simulink model "Diff_eqn"  (R2017b)
settings: Solver=VariableStepAuto  StartTime=0.0  StopTime=10.0  RelTol=1e-3
InitFcn:
  | A=2;
  |  B=4;
  |  C=200;
  | n=25;
  | Amp=10
undefined symbols (not defined in the file or in its folder): function_pulse
settings Model: Creator=ng8a07e  LastModifiedBy=ng8a07e

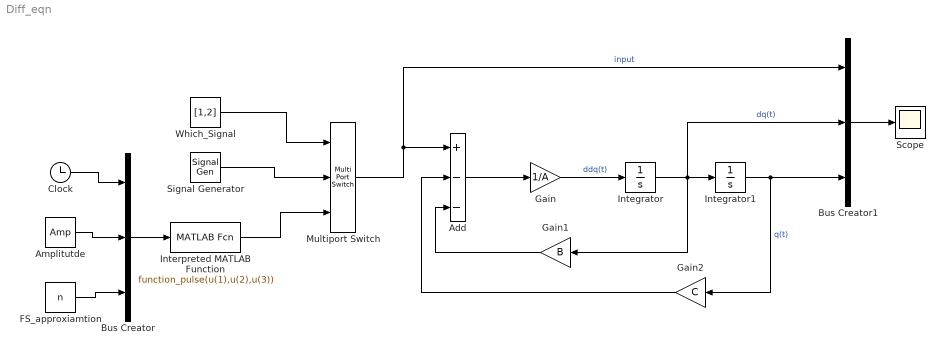
== system Diff_eqn ==
  Add : Sum  Inputs=+--
  Amplitutde : Constant  Value=Amp
  Bus Creator : BusCreator  Inputs=3
  Bus Creator1 : BusCreator  Inputs=3
  Clock : Clock
  FS_approxiamtion : Constant  Value=n
  Gain : Gain  Gain=1/A
  Gain1 : Gain  Gain=B
  Gain2 : Gain  Gain=C
  Integrator : Integrator
  Integrator1 : Integrator
  Interpreted MATLAB Function : MATLABFcn  MATLABFcn=function_pulse(u(1),u(2),u(3))
  Multiport Switch : MultiPortSwitch  Inputs=2
  Scope : Scope
  Signal Generator : SignalGenerator  WaveForm=square  Amplitude=-Amp/2  Frequency=3.15  Units=rad/sec
  Which_Signal : Constant  Value=[1,2]
  wires:
  Amplitutde/1 -> Bus Creator/2
  FS_approxiamtion/1 -> Bus Creator/3
  Clock/1 -> Bus Creator/1
  Bus Creator/1 -> Interpreted MATLAB Function/1
  Interpreted MATLAB Function/1 -> Multiport Switch/3
  Signal Generator/1 -> Multiport Switch/2
  Which_Signal/1 -> Multiport Switch/1
  Add/1 -> Gain/1
  Gain/1 -> Integrator/1  "ddq(t)"
  Integrator/1 -> Gain1/1, Bus Creator1/2, Integrator1/1  "dq(t)"
  Integrator1/1 -> Gain2/1, Bus Creator1/3  "q(t)"
  Multiport Switch/1 -> Add/1, Bus Creator1/1  "input"
  Gain1/1 -> Add/3
  Gain2/1 -> Add/2
  Bus Creator1/1 -> Scope/1
